simulink model "trackloop_3d_tb1"  (R2019b)
settings: Solver=FixedStepDiscrete  StartTime=0.0  StopTime=10000  RelTol=1e-3
values from neighbouring files (symbols this model uses):
  x1_dir = +1    (= 1)    [trackloop_3d_tb1_main.m]
  x1_init = x1mean - 2*x1sd    (= 0.8)    [trackloop_3d_tb1_main.m]
  x1_step = x1sd/10    (= 0.01)    [trackloop_3d_tb1_main.m]
  x1mag = 1    [trackloop_3d_tb1_main.m]
  x1mean = 1    [trackloop_3d_tb1_main.m]
  x1sd = .1    (= 0.1)    [trackloop_3d_tb1_main.m]
  x2_dir = +1    (= 1)    [trackloop_3d_tb1_main.m]
  x2_init = x2mean + 2*x2sd    (= 12)    [trackloop_3d_tb1_main.m]
  x2_step = x2sd/50    (= 0.02)    [trackloop_3d_tb1_main.m]
  x2mag = 1    [trackloop_3d_tb1_main.m]
  x2mean = 10    [trackloop_3d_tb1_main.m]
  x2sd = 1    [trackloop_3d_tb1_main.m]
  x3_dir = +1    (= 1)    [trackloop_3d_tb1_main.m]
  x3_init = x3mean - 5*x3sd    (= 50)    [trackloop_3d_tb1_main.m]
  x3_step = x3sd/5    (= 2)    [trackloop_3d_tb1_main.m]
  x3mag = 1    [trackloop_3d_tb1_main.m]
  x3mean = 100    [trackloop_3d_tb1_main.m]
  x3sd = 10    [trackloop_3d_tb1_main.m]
libraries: simulink x1, lib_dsphdlcontrol_v1 x1
settings Model: DataTypeOverride=Off  Creator=mbabst  LastModifiedBy=mbabst
settings DataIOCC: SaveOutput=off  SaveTime=off  ReturnWorkspaceOutputs=off
settings OptimizationCC: BlockReduction=off  ConditionallyExecuteInputs=off  DefaultParameterBehavior=Inlined  LifeSpan=inf
settings DebuggingCC: AlgebraicLoopMsg=error  SingleTaskRateTransMsg=error  StrictBusMsg=ErrorOnBusTreatedAsVector  SFUnexpectedBacktrackingDiag=warning  SFNoUnconditionalDefaultTransitionDiag=warning  ArithmeticOperatorsInVariantConditions=warning
settings HardwareCC: ProdBitPerPointer=32  ProdBitPerSizeT=32  ProdBitPerPtrDiffT=32  ProdLargestAtomicFloat=None  ProdIntDivRoundTo=Undefined  ProdEndianess=Unspecified  ProdWordSize=32  ProdHWDeviceType=ASIC/FPGA->ASIC/FPGA  ProdEqTarget=off
settings SFSimCC: SimUseLocalCustomCode=off  CustomCodeUndefinedFunction=UseInterfaceOnly
settings RTWCC: RTWUseLocalCustomCode=off
settings CodeAppCC: StateflowObjectComments=on
settings GRTTargetCC: TargetLangStandard=C89/C90 (ANSI)
settings ConfigComp: CovMetricSettings=dw  CovHtmlReporting=on  CovSaveCumulativeToWorkspaceVar=on  CovSaveSingleToWorkspaceVar=on  CovExternalEMLEnable=off

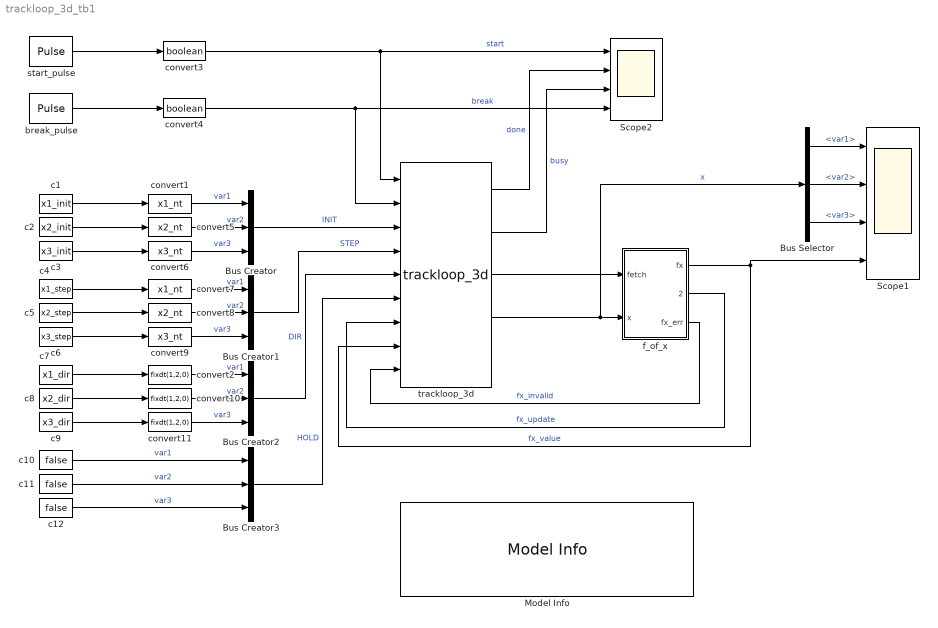
== system trackloop_3d_tb1 ==
  Bus Creator{,1..3} (4 alike) : BusCreator  Inputs=3
  Bus Selector : BusSelector  OutputSignals=var1,var2,var3
  Model Info : simulink/Model-Wide Utilities/Model Info  Frame=on  DisplayStringWithTags=|  HorizontalTextAlignment=Left  LeftAlignmentValue=0.02
      | Copyright (c) 2005-2021 DSPlogic, Inc.
      | Distributed under the terms of the Simplified BSD License.
      | The full license is in the file LICENSE, distributed with this software.
      | 
      | Model: %<ModelName> (v%<ModelVersion>)
      | Author: Michael Babst <mike.babst@dsplogic.com>
      | Created: by %<Creator> on %<Created>
      | Modified: by %<ModifiedBy> on %<LastModificationDate>
  Scope1 : Scope  NumInputPorts=4
  Scope2 : Scope  NumInputPorts=4
  break_pulse : DiscretePulseGenerator  Period=1e6  PhaseDelay=9000
  c1 : Constant  Value=x1_init  SampleTime=1
  c10 : Constant  Value=false  SampleTime=1
  c11 : Constant  Value=false  SampleTime=1
  c12 : Constant  Value=false  SampleTime=1
  c2 : Constant  Value=x2_init  SampleTime=1
  c3 : Constant  Value=x3_init  SampleTime=1
  c4 : Constant  Value=x1_step  SampleTime=1
  c5 : Constant  Value=x2_step  SampleTime=1
  c6 : Constant  Value=x3_step  SampleTime=1
  c7 : Constant  Value=x1_dir  SampleTime=1
  c8 : Constant  Value=x2_dir  SampleTime=1
  c9 : Constant  Value=x3_dir  SampleTime=1
  convert1 : DataTypeConversion  OutDataTypeStr=x1_nt
  convert10 : DataTypeConversion  OutDataTypeStr=fixdt(1,2,0)
  convert11 : DataTypeConversion  OutDataTypeStr=fixdt(1,2,0)
  convert2 : DataTypeConversion  OutDataTypeStr=fixdt(1,2,0)
  convert3 : DataTypeConversion  OutDataTypeStr=boolean
  convert4 : DataTypeConversion  OutDataTypeStr=boolean
  convert5 : DataTypeConversion  OutDataTypeStr=x2_nt
  convert6 : DataTypeConversion  OutDataTypeStr=x3_nt
  convert7 : DataTypeConversion  OutDataTypeStr=x1_nt
  convert8 : DataTypeConversion  OutDataTypeStr=x2_nt
  convert9 : DataTypeConversion  OutDataTypeStr=x3_nt
  f_of_x : Subsystem
  start_pulse : DiscretePulseGenerator  Period=1e6  PhaseDelay=5
  trackloop_3d : lib_dsphdlcontrol_v1/trackloop_3d  limit1=false  min1=0  max1=0  limit2=false  min2=0  max2=0  limit3=false  min3=0  max3=0
      settings: SourceProductName=DSPHDL Library
  wires:
  start_pulse/1 -> convert3/1
  break_pulse/1 -> convert4/1
  c1/1 -> convert1/1
  convert1/1 -> Bus Creator/1  "var1"
  trackloop_3d/3 -> f_of_x/1(fetch)
  trackloop_3d/4 -> Bus Selector/1, f_of_x/2(x)  "x"
  f_of_x/2(fx_valid) -> trackloop_3d/7  "fx_update"
  f_of_x/3(fx_err) -> trackloop_3d/9  "fx_invalid"
  convert3/1 -> trackloop_3d/1, Scope2/1  "start"
  convert4/1 -> Scope2/4, trackloop_3d/2  "break"
  Bus Creator/1 -> trackloop_3d/3  "INIT"
  convert5/1 -> Bus Creator/2  "var2"
  convert6/1 -> Bus Creator/3  "var3"
  c2/1 -> convert5/1
  c3/1 -> convert6/1
  c4/1 -> convert7/1
  convert7/1 -> Bus Creator1/1  "var1"
  convert8/1 -> Bus Creator1/2  "var2"
  convert9/1 -> Bus Creator1/3  "var3"
  c5/1 -> convert8/1
  c6/1 -> convert9/1
  Bus Creator1/1 -> trackloop_3d/4  "STEP"
  c7/1 -> convert2/1
  convert2/1 -> Bus Creator2/1  "var1"
  convert10/1 -> Bus Creator2/2  "var2"
  convert11/1 -> Bus Creator2/3  "var3"
  c8/1 -> convert10/1
  c9/1 -> convert11/1
  Bus Creator2/1 -> trackloop_3d/5  "DIR"
  Bus Selector/1 -> Scope1/1  "<var1>"
  Bus Selector/2 -> Scope1/2  "<var2>"
  Bus Selector/3 -> Scope1/3  "<var3>"
  f_of_x/1(fx) -> Scope1/4, trackloop_3d/8  "fx_value"
  trackloop_3d/1 -> Scope2/2  "done"
  trackloop_3d/2 -> Scope2/3  "busy"
  c10/1 -> Bus Creator3/1  "var1"
  c11/1 -> Bus Creator3/2  "var2"
  c12/1 -> Bus Creator3/3  "var3"
  Bus Creator3/1 -> trackloop_3d/6  "HOLD"

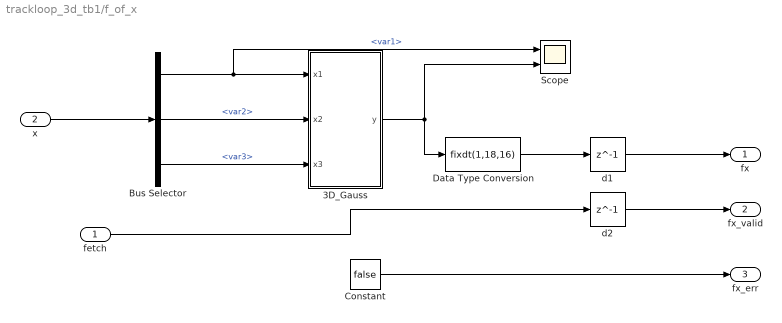
== system trackloop_3d_tb1/f_of_x ==
  fetch : Inport
  x : Inport  Port=2
  3D_Gauss : MATLAB Function  TreatAsAtomicUnit=on  mask{c1=x1mean, s1=x1sd, m1=x1mag, c2=x2mean, s2=x2sd, m2=x2mag, c3=x3mean, s3=x3sd, m3=x3mag}
      mask prompts: c1 "mean"; s1 "sd"; m1 "mag"; c2 "mean"; s2 "sd"; m2 "mag"; c3 "mean"; s3 "sd"; m3 "mag"
  Bus Selector : BusSelector  OutputSignals=var1,var2,var3
  Constant : Constant  Value=false  SampleTime=-1
  Data Type Conversion : DataTypeConversion  OutDataTypeStr=fixdt(1,18,16)
  Scope : Scope  NumInputPorts=2
  d1 : Delay  DelayLength=1  InitialCondition=0
  d2 : Delay  DelayLength=1  InitialCondition=0
  fx : Outport
  fx_valid : Outport  Port=2
  fx_err : Outport  Port=3
  wires:
  3D_Gauss/1(y) -> Data Type Conversion/1, Scope/2
  x/1 -> Bus Selector/1
  fetch/1 -> d2/1
  d1/1 -> fx/1
  d2/1 -> fx_valid/1
  Constant/1 -> fx_err/1
  Data Type Conversion/1 -> d1/1
  Bus Selector/1 -> Scope/1, 3D_Gauss/1(x1)  "<var1>"
  Bus Selector/2 -> 3D_Gauss/2(x2)  "<var2>"
  Bus Selector/3 -> 3D_Gauss/3(x3)  "<var3>"

== matlab function trackloop_3d_tb1/f_of_x/3D_Gauss ==
  data: x1 input; y output; x2 input; x3 input; c1 parameter; c2 parameter; c3 parameter; s1 parameter; s2 parameter; s3 parameter; m1 parameter; m2 parameter; m3 parameter
function y = fcn(x1,x2,x3, c1, c2, c3, s1, s2, s3, m1, m2, m3)
%#codegen

%% 3D Gaussian function
fx1 = m1 * exp((-(double(x1) - c1).^2)./(2*s1^2));
fx2 = m2 * exp((-(double(x2) - c2).^2)./(2*s2^2));
fx3 = m3 * exp((-(double(x3) - c3).^2)./(2*s3^2));
y = fx1.*fx2.*fx3;
